simulink model "BMS_Arch"  (R2022b)
settings: configuration reference "BMS_Sw_CodeGenConfig" (kept outside this file)
model workspace: external: MAT-File H:\0\New MAAM\10 - MBD\Battary Management System\SWE.3 CDD\DataTypes\Data_Script.mat (data not in the file)
undefined symbols (not defined in the file): BATT
settings Model: DataDictionary=BMS_Arch_DD.sldd  EnableAccessToBaseWorkspace=off  Creator=MAAM  LastModifiedBy=MAAM
settings ConfigSetRef: SourceName=BMS_Sw_CodeGenConfig

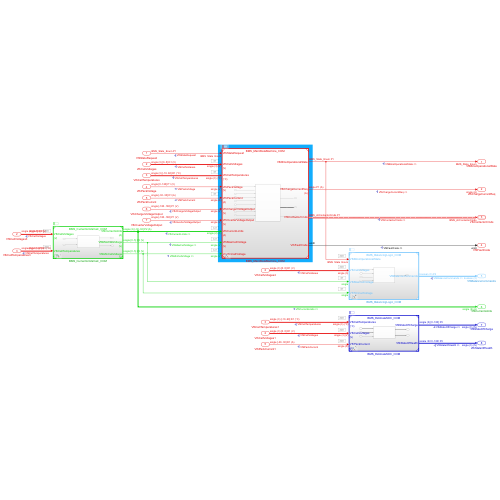
[thumbnail: Simulink's stored preview of the top-level diagram]
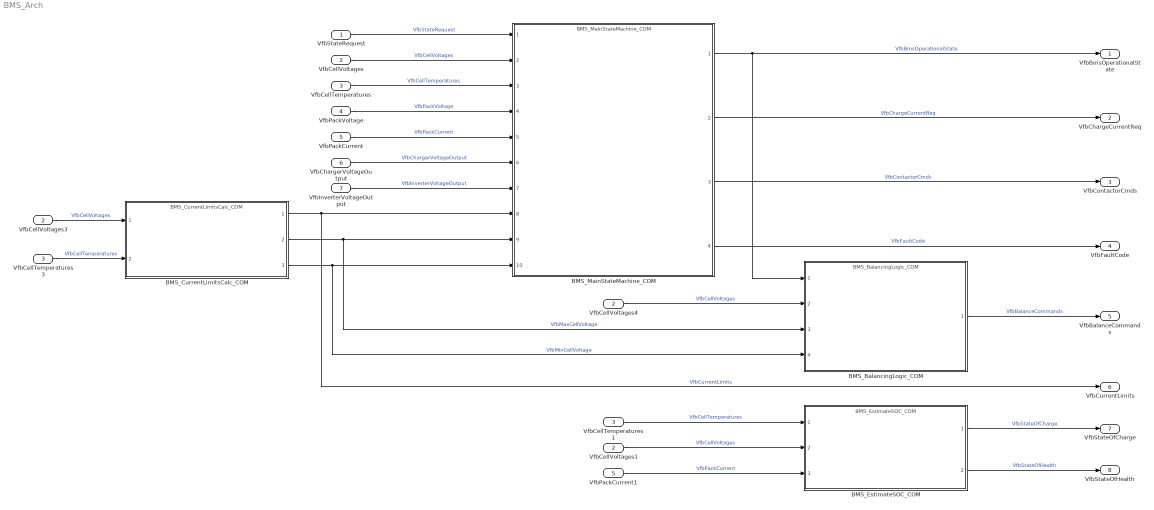
== system BMS_Arch ==
  VfbStateRequest : Inport  OutDataTypeStr=Enum: BMS_State_Enum  PortDimensions=1
  VfbCellVoltages : Inport  Port=2  OutDataTypeStr=single  Unit=V  PortDimensions=BATT.Package.NumModules
  VfbCellTemperatures : Inport  Port=3  OutDataTypeStr=single  Unit=°C  PortDimensions=BATT.Package.NumModules
  VfbPackVoltage : Inport  Port=4  OutDataTypeStr=single  Unit=V  PortDimensions=1
  VfbPackCurrent : Inport  Port=5  OutDataTypeStr=single  Unit=A  PortDimensions=1
  VfbChargerVoltageOutput : Inport  Port=6  OutDataTypeStr=single  Unit=V  PortDimensions=1
  VfbInverterVoltageOutput : Inport  Port=7  OutDataTypeStr=single  Unit=V  PortDimensions=1
  BMS_BalancingLogic_COM : ModelReference  ModelNameDialog=BMS_BalancingLogic_COM.slx  SimulationMode=Normal  ScheduleRates=on  ScheduleRatesWith=Schedule Editor  HasExplicitPartitions=on  ModelReferenceVersion=1.53
  BMS_CurrentLimitsCalc_COM : ModelReference  ModelNameDialog=BMS_CurrentLimitsCalc_COM.slx  SimulationMode=Normal  ScheduleRates=on  ScheduleRatesWith=Schedule Editor  HasExplicitPartitions=on  ModelReferenceVersion=1.46
  BMS_EstimateSOC_COM : ModelReference  ModelNameDialog=BMS_EstimateSOC_COM.slx  SimulationMode=Normal  ScheduleRates=on  ScheduleRatesWith=Schedule Editor  HasExplicitPartitions=on  ModelReferenceVersion=1.41
  BMS_MainStateMachine_COM : ModelReference  ModelNameDialog=BMS_MainStateMachine_COM.slx  SimulationMode=Normal  ScheduleRates=on  ScheduleRatesWith=Schedule Editor  HasExplicitPartitions=on  ModelReferenceVersion=1.83
  VfbCellTemperatures1 : InportShadow  Port=3  OutDataTypeStr=single  Unit=°C  PortDimensions=BATT.Package.NumModules
  VfbCellTemperatures3 : InportShadow  Port=3  OutDataTypeStr=single  Unit=°C  PortDimensions=BATT.Package.NumModules
  VfbCellVoltages1 : InportShadow  Port=2  OutDataTypeStr=single  Unit=V  PortDimensions=BATT.Package.NumModules
  VfbCellVoltages3 : InportShadow  Port=2  OutDataTypeStr=single  Unit=V  PortDimensions=BATT.Package.NumModules
  VfbCellVoltages4 : InportShadow  Port=2  OutDataTypeStr=single  Unit=V  PortDimensions=BATT.Package.NumModules
  VfbPackCurrent1 : InportShadow  Port=5  OutDataTypeStr=single  Unit=A  PortDimensions=1
  VfbBmsOperationalState : Outport  OutDataTypeStr=Enum: BMS_State_Enum  PortDimensions=1
  VfbChargeCurrentReq : Outport  Port=2  OutDataTypeStr=single  Unit=A  PortDimensions=1
  VfbContactorCmds : Outport  Port=3  OutDataTypeStr=Bus: BMS_strContactorCmds  BusOutputAsStruct=on
  VfbFaultCode : Outport  Port=4  OutDataTypeStr=uint8  PortDimensions=1
  VfbBalanceCommands : Outport  Port=5  OutDataTypeStr=boolean  PortDimensions=BATT.Package.Ns_Module*BATT.Package.NumModules
  VfbCurrentLimits : Outport  Port=6  OutDataTypeStr=single  Unit=A
  VfbStateOfCharge : Outport  Port=7  OutDataTypeStr=single  Unit=%
  VfbStateOfHealth : Outport  Port=8  OutDataTypeStr=single  Unit=%
  wires:
  BMS_CurrentLimitsCalc_COM/2 -> BMS_MainStateMachine_COM/9, BMS_BalancingLogic_COM/3  "VfbMaxCellVoltage"
  BMS_CurrentLimitsCalc_COM/3 -> BMS_BalancingLogic_COM/4, BMS_MainStateMachine_COM/10  "VfbMinCellVoltage"
  VfbStateRequest/1 -> BMS_MainStateMachine_COM/1  "VfbStateRequest"
  VfbCellVoltages/1 -> BMS_MainStateMachine_COM/2  "VfbCellVoltages"
  VfbCellTemperatures/1 -> BMS_MainStateMachine_COM/3  "VfbCellTemperatures"
  VfbPackVoltage/1 -> BMS_MainStateMachine_COM/4  "VfbPackVoltage"
  VfbPackCurrent/1 -> BMS_MainStateMachine_COM/5  "VfbPackCurrent"
  VfbChargerVoltageOutput/1 -> BMS_MainStateMachine_COM/6  "VfbChargerVoltageOutput"
  VfbInverterVoltageOutput/1 -> BMS_MainStateMachine_COM/7  "VfbInverterVoltageOutput"
  VfbCellTemperatures3/1 -> BMS_CurrentLimitsCalc_COM/2  "VfbCellTemperatures"
  BMS_MainStateMachine_COM/2 -> VfbChargeCurrentReq/1  "VfbChargeCurrentReq"
  BMS_MainStateMachine_COM/1 -> BMS_BalancingLogic_COM/1, VfbBmsOperationalState/1  "VfbBmsOperationalState"
  BMS_BalancingLogic_COM/1 -> VfbBalanceCommands/1  "VfbBalanceCommands"
  BMS_CurrentLimitsCalc_COM/1 -> BMS_MainStateMachine_COM/8, VfbCurrentLimits/1  "VfbCurrentLimits"
  VfbPackCurrent1/1 -> BMS_EstimateSOC_COM/3  "VfbPackCurrent"
  VfbCellVoltages1/1 -> BMS_EstimateSOC_COM/2  "VfbCellVoltages"
  VfbCellTemperatures1/1 -> BMS_EstimateSOC_COM/1  "VfbCellTemperatures"
  VfbCellVoltages3/1 -> BMS_CurrentLimitsCalc_COM/1  "VfbCellVoltages"
  VfbCellVoltages4/1 -> BMS_BalancingLogic_COM/2  "VfbCellVoltages"
  BMS_EstimateSOC_COM/1 -> VfbStateOfCharge/1  "VfbStateOfCharge"
  BMS_EstimateSOC_COM/2 -> VfbStateOfHealth/1  "VfbStateOfHealth"
  BMS_MainStateMachine_COM/3 -> VfbContactorCmds/1  "VfbContactorCmds"
  BMS_MainStateMachine_COM/4 -> VfbFaultCode/1  "VfbFaultCode"
